simulink model "lab2"  (R2017a)
settings: Solver=FixedStepAuto  StartTime=0.0  StopTime=2  FixedStep=1e-7  RelTol=1e-3
libraries: dspstat3 x1, simulink x1
settings Model: Creator=chris  LastModifiedBy=chris

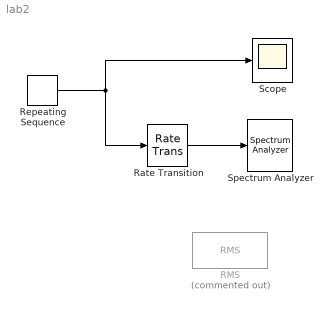
== system lab2 ==
  RMS : dspstat3/RMS  Commented=on  run=off  directionMode=Each column  dimension=1  InputProcessing=Columns as channels (frame based)  reset_popup=None
  Rate Transition : RateTransition
  Repeating Sequence : simulink/Sources/Repeating Sequence  rep_seq_t=[0:1e-7:7e-4 7e-4+1e-7:1e-7:9e-4 9e-4+1e-7:1e-7:1e-3]  rep_seq_y=[2857.1428571429*(0:1e-7:7e-4) 7e-4+1e-7:1e-7:9e-4 (-20000*(9e-4+1e-7:1e-7:1e-3)+18)]
  Scope : Scope
  Spectrum Analyzer : SpectrumAnalyzer
  wires:
  Repeating Sequence/1 -> Scope/1, Rate Transition/1
  Rate Transition/1 -> Spectrum Analyzer/1
